simulink model "pwm_avg_controlled_system"  (R2017a)
settings: Solver=FixedStepAuto  StartTime=0.0  StopTime=t_f  FixedStep=1e-6  RelTol=1e-3
values from neighbouring files (symbols this model uses):
  A = double(subs(A, symbs, vals))    [load_params.m]    (also in main.m)
  B = double(subs(B, symbs, vals))    [load_params.m]    (also in main.m)
  C = sysd.c    [load_discrete_pred_controller.m]    (also in load_params.m = double(subs(C, symbs, vals)); load_pwm_avg_pred_controller.m; main.m = double(subs(C, symbs, vals)))
  Ts_val = 1.1e-2    (= 0.011)    [ss_value.m]
  x0 = [0; 0; 0]    [main.m]    (also in sim_controlled_system.m = [0; 0]; sim_system.m)
undefined symbols (not defined in the file or in its folder): Ctilde, torque_ref, Vcc_val
settings Model: Creator=brunolnetto  LastModifiedBy=brunolnetto
settings SolverCC: AlgebraicLoopSolver=LineSearch

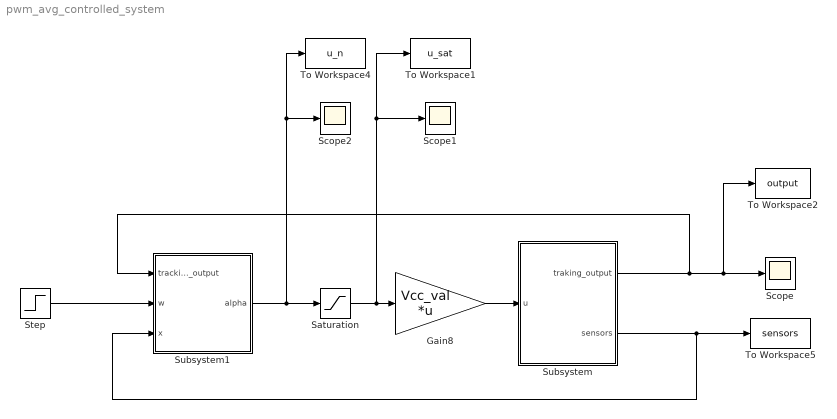
== system pwm_avg_controlled_system ==
  Gain8 : Gain  Gain=Vcc_val  Multiplication=Matrix(K*u) (u vector)
  Saturation : Saturate  UpperLimit=1  LowerLimit=-1
  Scope : Scope
  Scope1 : Scope
  Scope2 : Scope
  Step : Step  Time=0  After=torque_ref  SampleTime=Ts_val
  Subsystem : Subsystem
  Subsystem1 : Subsystem
  To Workspace1 : ToWorkspace  VariableName=u_sat  SaveFormat=Structure With Time  SampleTime=-1
  To Workspace2 : ToWorkspace  VariableName=output  SaveFormat=Structure With Time  SampleTime=-1
  To Workspace4 : ToWorkspace  VariableName=u_n  SaveFormat=Structure With Time  SampleTime=-1
  To Workspace5 : ToWorkspace  VariableName=sensors  SaveFormat=Structure With Time  SampleTime=-1
  wires:
  Subsystem/1(traking_output) -> To Workspace2/1, Scope/1, Subsystem1/1(tracking_output)
  Subsystem/2(sensors) -> To Workspace5/1, Subsystem1/3(x)
  Step/1 -> Subsystem1/2(w)
  Saturation/1 -> Scope1/1, To Workspace1/1, Gain8/1
  Subsystem1/1(alpha) -> Scope2/1, To Workspace4/1, Saturation/1
  Gain8/1 -> Subsystem/1(u)

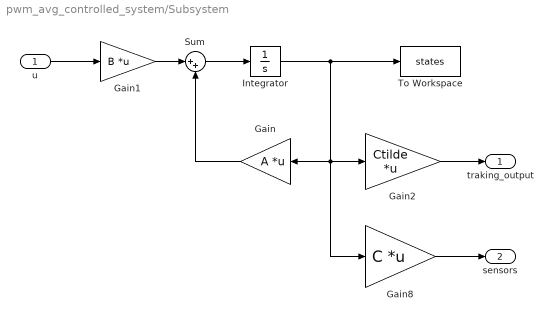
== system pwm_avg_controlled_system/Subsystem ==
  u : Inport
  Gain : Gain  Gain=A  Multiplication=Matrix(K*u) (u vector)
  Gain1 : Gain  Gain=B  Multiplication=Matrix(K*u) (u vector)
  Gain2 : Gain  Gain=Ctilde  Multiplication=Matrix(K*u) (u vector)
  Gain8 : Gain  Gain=C  Multiplication=Matrix(K*u) (u vector)
  Integrator : Integrator  InitialCondition=x0
  Sum : Sum  Inputs=|++
  To Workspace : ToWorkspace  VariableName=states  SaveFormat=Structure With Time  SampleTime=-1
  traking_output : Outport
  sensors : Outport  Port=2
  wires:
  Gain8/1 -> sensors/1
  Gain1/1 -> Sum/1
  Integrator/1 -> To Workspace/1, Gain2/1, Gain8/1, Gain/1
  u/1 -> Gain1/1
  Gain/1 -> Sum/2
  Sum/1 -> Integrator/1
  Gain2/1 -> traking_output/1

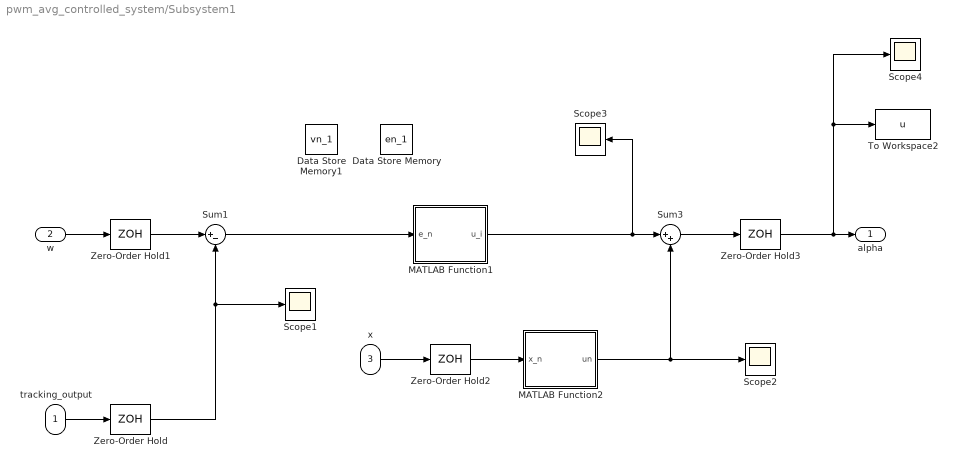
== system pwm_avg_controlled_system/Subsystem1 ==
  tracking_output : Inport
  w : Inport  Port=2
  x : Inport  Port=3
  Data Store Memory : DataStoreMemory  DataStoreName=en_1  ReadBeforeWriteMsg=warning  WriteAfterWriteMsg=warning  WriteAfterReadMsg=warning  InitialValue=e0  ShowAdditionalParam=off  OutDataTypeStr=double
  Data Store Memory1 : DataStoreMemory  DataStoreName=vn_1  ReadBeforeWriteMsg=warning  WriteAfterWriteMsg=warning  WriteAfterReadMsg=warning  ShowAdditionalParam=off  OutDataTypeStr=double
  MATLAB Function1 : MATLAB Function  TreatAsAtomicUnit=on
  MATLAB Function2 : MATLAB Function  TreatAsAtomicUnit=on
  Scope{1..4} (4 alike) : Scope
  Sum1 : Sum  Inputs=|+-
  Sum3 : Sum  Inputs=|++
  To Workspace2 : ToWorkspace  VariableName=u  SaveFormat=Structure With Time  SampleTime=-1
  Zero-Order Hold{,1..3} (4 alike) : ZeroOrderHold  SampleTime=Ts_val
  alpha : Outport
  wires:
  Zero-Order Hold1/1 -> Sum1/1
  tracking_output/1 -> Zero-Order Hold/1
  Zero-Order Hold2/1 -> MATLAB Function2/1(x_n)
  x/1 -> Zero-Order Hold2/1
  Sum1/1 -> MATLAB Function1/1(e_n)
  Zero-Order Hold/1 -> Scope1/1, Sum1/2
  w/1 -> Zero-Order Hold1/1
  MATLAB Function2/1(un) -> Sum3/2, Scope2/1
  MATLAB Function1/1(u_i) -> Scope3/1, Sum3/1
  Sum3/1 -> Zero-Order Hold3/1
  Zero-Order Hold3/1 -> Scope4/1, To Workspace2/1, alpha/1

== matlab function pwm_avg_controlled_system/Subsystem1/MATLAB Function1 ==
  data: e_n input; u_i output; en_1 data_store_memory; vn_1 data_store_memory; params parameter
function u_i = integrator(e_n, params)
    global vn_1;
    global en_1;
    
    v_n = vn_1 + en_1 ;
    
    u_i = params.Ki*v_n;
    
    en_1 = e_n;
    vn_1 = v_n;
end

== matlab function pwm_avg_controlled_system/Subsystem1/MATLAB Function2 ==
  data: x_n input; un output; en_1 data_store_memory; vn_1 data_store_memory; params parameter
function un = proportional(x_n, params)
    un = - params.Kp*x_n;
end
